simulink model "MSE452_PV_Project_Model_Student_R2018b"  (Simulink 9.2)
settings: Solver=ode45  StartTime=0.0  StopTime=0.5  MaxStep=1e-4  RelTol=1e-3
values from neighbouring files (symbols this model uses):
  Cdc = 3*Cb_solar    [MSE452_PV_Project_Model_Parameters_Student.m]    (also in MSE452_PV_Project_Model_Parameters_Studentv2.m; MSE452_PV_Project_Model_Parameters_Studentv3.m)
  Cpv = 0.05*Cb_solar    [MSE452_PV_Project_Model_Parameters_Student.m]    (also in MSE452_PV_Project_Model_Parameters_Studentv2.m; MSE452_PV_Project_Model_Parameters_Studentv3.m)
  Fb = 60    [MSE452_PV_Project_Model_Parameters_Student.m]    (also in MSE452_PV_Project_Model_Parameters_Studentv2.m; MSE452_PV_Project_Model_Parameters_Studentv3.m)
  Fs_boost = 10000    [MSE452_PV_Project_Model_Parameters_Student.m]    (also in MSE452_PV_Project_Model_Parameters_Studentv2.m; MSE452_PV_Project_Model_Parameters_Studentv3.m)
  Fsampling = 10e3    (= 10000)    [MSE452_PV_Project_Model_Parameters_Student.m]    (also in MSE452_PV_Project_Model_Parameters_Studentv2.m; MSE452_PV_Project_Model_Parameters_Studentv3.m)
  Lboost = 0.5*Lb_solar    [MSE452_PV_Project_Model_Parameters_Student.m]    (also in MSE452_PV_Project_Model_Parameters_Studentv2.m; MSE452_PV_Project_Model_Parameters_Studentv3.m)
  Lgrid = Lgrid_pu*Lb_solar    [MSE452_PV_Project_Model_Parameters_Student.m]    (also in MSE452_PV_Project_Model_Parameters_Studentv2.m; MSE452_PV_Project_Model_Parameters_Studentv3.m)
  Lgrid_pu = 0.2    [MSE452_PV_Project_Model_Parameters_Student.m]    (also in MSE452_PV_Project_Model_Parameters_Studentv2.m; MSE452_PV_Project_Model_Parameters_Studentv3.m)
  Rgrid = Rgrid_pu*Zb_solar    [MSE452_PV_Project_Model_Parameters_Student.m]    (also in MSE452_PV_Project_Model_Parameters_Studentv2.m; MSE452_PV_Project_Model_Parameters_Studentv3.m)
  Vb = 208/sqrt(3)    [MSE452_PV_Project_Model_Parameters_Student.m]    (also in MSE452_PV_Project_Model_Parameters_Studentv2.m; MSE452_PV_Project_Model_Parameters_Studentv3.m)
  Vdc_ref = sqrt(6)*(1/1)    [MSE452_PV_Project_Model_Parameters_Student.m]    (also in MSE452_PV_Project_Model_Parameters_Studentv2.m; MSE452_PV_Project_Model_Parameters_Studentv3.m = 2.44949)
undefined symbols (not defined in the file or in its folder): Rdc
undefined symbols (not defined in the file): Fs_inv, Ib_solar
libraries: powerlib x19, simulink x4, powerlib_extras x3, simulink_extras x2, re_lib x1, eePwmGenerator x1
settings Model: Creator=Student  LastModifiedBy=dw
settings SolverCC: ZeroCrossAlgorithm=Adaptive  AlgebraicLoopSolver=LineSearch
settings DataIOCC: LimitDataPoints=off  SaveFormat=Dataset  SignalLoggingSaveFormat=Dataset
settings DebuggingCC: UnderspecifiedInitializationDetection=Simplified  MergeDetectMultiDrivingBlocksExec=error  FcnCallInpInsideContextMsg=error  StateNameClashWarn=none  SFUnexpectedBacktrackingDiag=error  SFNoUnconditionalDefaultTransitionDiag=error  SFExecutionAtInitializationDiag=warning
settings HardwareCC: ProdBitPerPointer=64  ProdLargestAtomicFloat=Float  ProdIntDivRoundTo=Zero  ProdEndianess=LittleEndian  ProdHWDeviceType=Specified
settings ModelReferenceCC: PropagateSignalLabelsOutOfModel=on
settings GRTTargetCC: TargetLangStandard=C99 (ISO)  CombineOutputUpdateFcns=on  GRTInterface=off
settings ConfigComp: CovMetricSettings=dwe  CovSaveCumulativeToWorkspaceVar=off  CovSaveSingleToWorkspaceVar=off  CovExternalEMLEnable=on
settings SimscapeCC: SimscapeNormalizeSystem=off

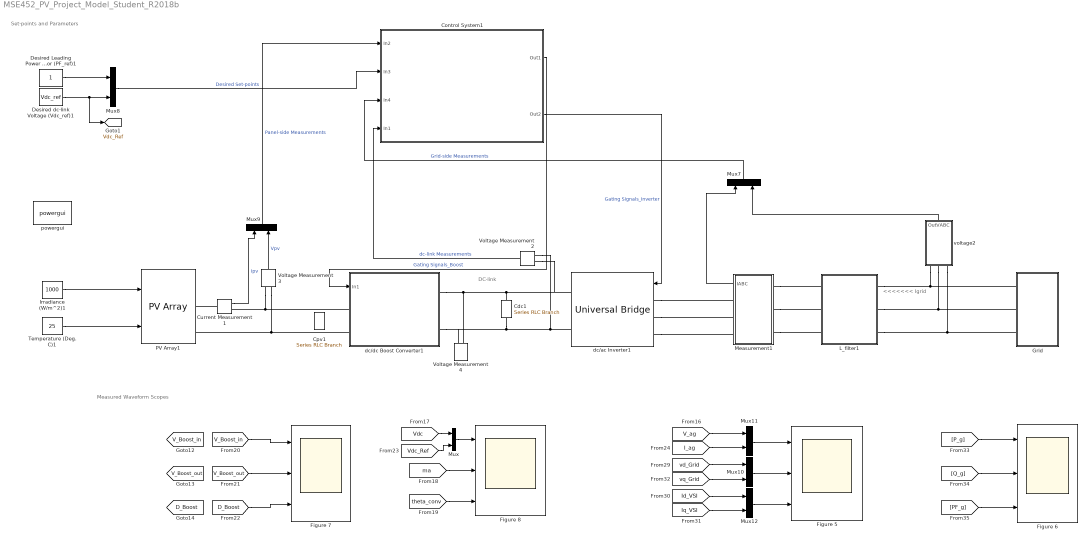
== system MSE452_PV_Project_Model_Student_R2018b ==
  note: DC-link
  note: Set-points and Parameters
  note: <<<<<<< Igrid
  note: Measured Waveform Scopes
  " voltage2" : Subsystem  mask{Base=Vb}
      mask prompts: Base "Base value"
  Cdc1 : powerlib/Elements/Series RLC Branch  LConnTagsString=__new0  RConnTagsString=__new0  BranchType=C  Resistance=Rdc  Inductance=1e-3  SetiL0=off  InitialCurrent=0  Capacitance=Cdc  Setx0=on  InitialVoltage=Vdc_capacitor_initial  Measurements=None
  Control System1 : Subsystem
  Cpv1 : powerlib/Elements/Series RLC Branch  LConnTagsString=__new0  RConnTagsString=__new0  BranchType=C  Resistance=Rdc  Inductance=1e-3  SetiL0=off  InitialCurrent=0  Capacitance=Cpv  Setx0=off  InitialVoltage=Vdc_capacitor_initial  Measurements=None
  Current Measurement1 : powerlib/Measurements/Current Measurement  PhasorSimulation=off  OutputType=Complex  PSBequivalent=0
  Desired Leading Power Factor (PF_ref)1 : Constant
  Desired dc-link Voltage (Vdc_ref)1 : Constant  Value=Vdc_ref
  Figure {5..8} (4 alike) : Scope  NumInputPorts=3
  Grid : Subsystem
  Irradiance (W/m^2)1 : Constant  Value=1000
  L_filter1 : Subsystem
  Measurement1 : Subsystem  mask{Base=Ib_solar}
      mask prompts: Base "Base value"
  Mux{,7..12} (7 alike) : Mux  Inputs=2
  PV Array1 : re_lib/Solar/PV Array  Npar=8  Nser=5  PlotType=array @ 1000 W/m2 & specified temperatures  S_vec="[ 1000 800 600 400 200  ]"  Temp_C_vec="[ 55 25  ]"  ModuleName=User-defined  PlotWhenSelected=off  Pm=229.89  Ncell=60  Voc=36.7  Isc=8.4  Vm=29.1  Im=7.9  beta_Voc_pc=-0.33899  alpha_Isc_pc=0.124  beta_Voc=-0.12441  alpha_Isc=0.010416  IL=8.4691  I0=1.485e-10  nI=0.96205  Rsh=216.9373  Rs=0.41347  RobustModel=off  RobustCellTemperature=25  BAL=off  Tc=1e-6  Tfilter=5e-5
  Temperature (Deg. C)1 : Constant  Value=25
  Voltage Measurement2 : powerlib/Measurements/Voltage Measurement  PhasorSimulation=off  OutputType=Complex  PSBequivalent=0
  Voltage Measurement3 : powerlib/Measurements/Voltage Measurement  PhasorSimulation=off  OutputType=Complex  PSBequivalent=0
  Voltage Measurement4 : powerlib/Measurements/Voltage Measurement  PhasorSimulation=off  OutputType=Complex  PSBequivalent=0
  dc/ac Inverter1 : powerlib/Power Electronics/Universal Bridge  Arms=3  SnubberResistance=1e5  SnubberCapacitance=inf  Device=IGBT / Diodes  Ron=1e-6  Lon=0  ForwardVoltages="[  0  0  ]"  ForwardVoltage=0  GTOparameters=[ 10e-6 , 20e-6 ]  IGBTparameters=[ 1e-6 , 2e-6 ]  Measurements=None  Measurements_2=None  converterType=Rectifier
  dc/dc Boost Converter1 : Subsystem
  powergui : powerlib/powergui  Priority=1  SimulationMode=Discrete  SampleTime=1e-6  frequency=60  Iterations=50  frequencyindice=0  Pbase=100e6  ErrMax=1e-4  UnitsV=kV  UnitsW=MW  buscounter=0  FunctionMessages=off  echomessages=off  EnableUseOfTLC=off  CurrentSourceSwitches=off  DisableSnubberDevices=off  DisableRonSwitches=off  DisableVfSwitches=off  DisplayEquations=off  AutomaticDiscreteSolvers=off  SolverType=Tustin  Interpol=off  ExternalGateDelay=off  methode=off  Ts=100  x0status=blocks  SPID=on  SwTol=0  HookPort=off  NonlinearTolerance=1e-4  nMaxIteration=100  ContinueOnMaxIteration=off  RestoreLinks=warning  ResistiveCurrentMeasurement=off  Frange=[0:2:500]  Ylog=off  Xlog=on  ShowGrid=off  save=off  variable=ZData  structure=0  ZoomFFT=off  StartTime=0.0  cycles=1  DisplayStyle=1  fundamental=60  FreqAxis=off  MaxFrequency=1000  frequencyindicesteady=1  RmsSteady=1  display=off
  tag scope: D_Boost=global, V_Boost_in=global, V_Boost_out=global, Vdc_Ref=global
  wires:
  [PF_g] -> Figure 6/3
  [Q_g] -> Figure 6/2
  Mux8/1 -> Control System1/2(In3)  "Desired Set-points"
  [vd_Grid] -> Mux10/1
  [V_ag] -> Mux11/1
  Control System1/1(Out1) -> dc/dc Boost Converter1/1(In1)  "Gating Signals_Boost"
  [P_g] -> Figure 6/1
  Mux/1 -> Figure 8/1
  [theta_conv] -> Figure 8/3
  Mux10/1 -> Figure 5/2
  [Id_VSI] -> Mux12/1
  Mux7/1 -> Control System1/3(In4)  "Grid-side Measurements"
  [V_Boost_out] -> Figure 7/2
  [Vdc_Ref] -> Mux/2
  Mux12/1 -> Figure 5/3
  Voltage Measurement2/1 -> Control System1/4(In1)  "dc-link Measurements"
  Desired Leading Power Factor (PF_ref)1/1 -> Mux8/1
  Irradiance (W/m^2)1/1 -> PV Array1/1
  [vq_Grid] -> Mux10/2
  [Iq_VSI] -> Mux12/2
  Mux9/1 -> Control System1/1(In2)  "Panel-side Measurements"
  Temperature (Deg. C)1/1 -> PV Array1/2
  [Vdc] -> Mux/1
  [V_Boost_in] -> Figure 7/1
  Current Measurement1/1 -> Mux9/1  "Ipv"
  [I_ag] -> Mux11/2
  [ma] -> Figure 8/2
  Mux11/1 -> Figure 5/1
  " voltage2"/1(OutVABC) -> Mux7/2
  Desired dc-link Voltage (Vdc_ref)1/1 -> [Vdc_Ref], Mux8/2
  [D_Boost] -> Figure 7/3
  Voltage Measurement3/1 -> Mux9/2  "Vpv"
  Measurement1/1(IABC) -> Mux7/1
  Control System1/2(Out2) -> dc/ac Inverter1/1  "Gating Signals_Inverter"
  connections:
  dc/dc Boost Converter1/LConn2 -- PV Array1/RConn2 -- Voltage Measurement3/LConn2
  dc/ac Inverter1/RConn2 -- Voltage Measurement2/LConn2 -- Cdc1/RConn1 -- dc/dc Boost Converter1/RConn2 -- Voltage Measurement4/LConn2
  L_filter1/LConn1 -- Grid/RConn1 -- " voltage2"/LConn1
  Voltage Measurement4/LConn1 -- dc/dc Boost Converter1/RConn1 -- Cdc1/LConn1 -- Voltage Measurement2/LConn1 -- dc/ac Inverter1/RConn1
  L_filter1/LConn3 -- Grid/RConn3 -- " voltage2"/LConn3
  L_filter1/LConn2 -- Grid/RConn2 -- " voltage2"/LConn2
  dc/dc Boost Converter1/LConn1 -- Current Measurement1/RConn1 -- Voltage Measurement3/LConn1
  Current Measurement1/LConn1 -- PV Array1/RConn1
  Measurement1/LConn3 -- L_filter1/RConn3
  Measurement1/LConn1 -- L_filter1/RConn1
  Measurement1/LConn2 -- L_filter1/RConn2
  dc/ac Inverter1/LConn1 -- Measurement1/RConn1
  dc/ac Inverter1/LConn3 -- Measurement1/RConn3
  dc/ac Inverter1/LConn2 -- Measurement1/RConn2

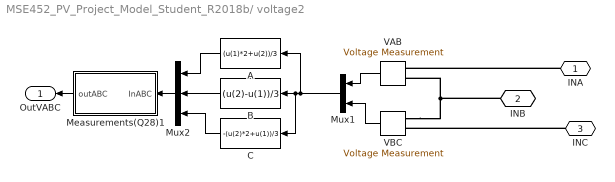
== system MSE452_PV_Project_Model_Student_R2018b/ voltage2 ==
  A : Fcn  Expr=(u(1)*2+u(2))/3
  B : Fcn  Expr=(u(2)-u(1))/3
  C : Fcn  Expr=-(u(2)*2+u(1))/3
  Measurements(Q28)1 : Subsystem  mask{Base=Base}
      mask prompts: Base "Base Value"
  Mux1 : Mux  Inputs=2
  Mux2 : Mux  Inputs=3
  VAB : powerlib/Measurements/Voltage Measurement  PhasorSimulation=off  OutputType=Complex  PSBequivalent=0
  VBC : powerlib/Measurements/Voltage Measurement  PhasorSimulation=off  OutputType=Complex  PSBequivalent=0
  INA : PMIOPort  Side=Left
  INB : PMIOPort  Port=2  Side=Left
  INC : PMIOPort  Port=3  Side=Left
  OutVABC : Outport  VectorParamsAs1DForOutWhenUnconnected=off
  wires:
  Measurements(Q28)1/1(outABC) -> OutVABC/1
  VAB/1 -> Mux1/1
  VBC/1 -> Mux1/2
  Mux1/1 -> B/1, C/1, A/1
  A/1 -> Mux2/1
  B/1 -> Mux2/2
  Mux2/1 -> Measurements(Q28)1/1(InABC)
  C/1 -> Mux2/3
  connections:
  VBC/LConn1 -- VAB/LConn2 -- INB/RConn1
  INC/RConn1 -- VBC/LConn2
  INA/RConn1 -- VAB/LConn1

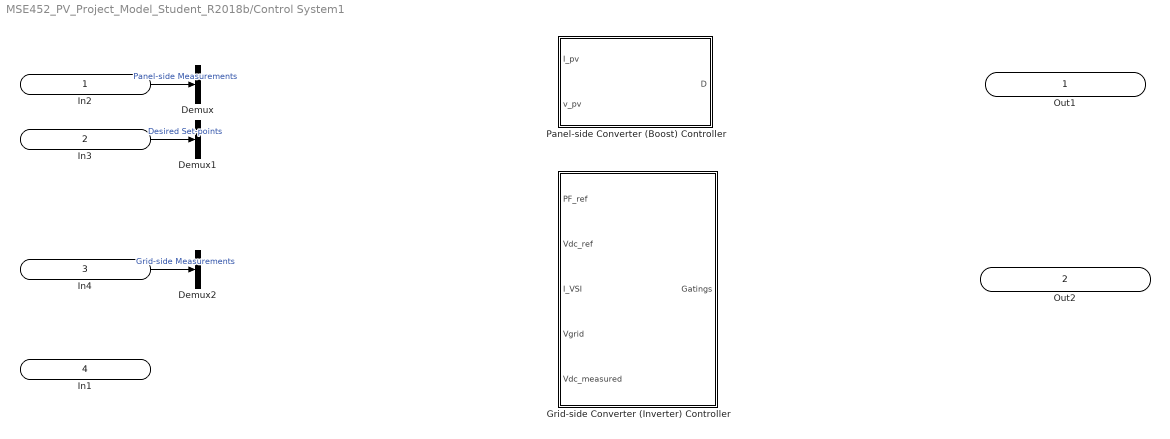
== system MSE452_PV_Project_Model_Student_R2018b/Control System1 ==
  In2 : Inport
  In3 : Inport  Port=2
  In4 : Inport  Port=3
  In1 : Inport  Port=4
  Demux : Demux  Outputs=2
  Demux1 : Demux  Outputs=2
  Demux2 : Demux  Outputs=2
  Grid-side Converter (Inverter) Controller : Subsystem
  Panel-side Converter (Boost) Controller : Subsystem
  Out1 : Outport  VectorParamsAs1DForOutWhenUnconnected=off
  Out2 : Outport  Port=2  VectorParamsAs1DForOutWhenUnconnected=off
  wires:
  In2/1 -> Demux/1  "Panel-side Measurements"
  In3/1 -> Demux1/1  "Desired Set-points"
  In4/1 -> Demux2/1  "Grid-side Measurements"

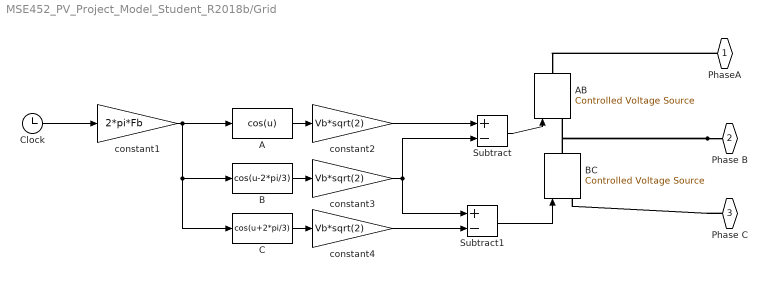
== system MSE452_PV_Project_Model_Student_R2018b/Grid ==
  A : Fcn  Expr=cos(u)
  AB : powerlib/Electrical Sources/Controlled Voltage Source  Initialize=off  Source_Type=AC  Amplitude=0  Phase=0  Frequency=0  Measurements=None
  B : Fcn  Expr=cos(u-2*pi/3)
  BC : powerlib/Electrical Sources/Controlled Voltage Source  Initialize=off  Source_Type=AC  Amplitude=0  Phase=0  Frequency=0  Measurements=None
  C : Fcn  Expr=cos(u+2*pi/3)
  Clock : Clock
  Subtract : Sum  Inputs=+-
  Subtract1 : Sum  Inputs=+-
  constant1 : Gain  Gain=2*pi*Fb
  constant2 : Gain  Gain=Vb*sqrt(2)
  constant3 : Gain  Gain=Vb*sqrt(2)
  constant4 : Gain  Gain=Vb*sqrt(2)
  PhaseA : PMIOPort  Side=Right
  Phase B : PMIOPort  Port=2  Side=Right
  Phase C : PMIOPort  Port=3  Side=Right
  wires:
  Subtract/1 -> AB/1
  Subtract1/1 -> BC/1
  A/1 -> constant2/1
  B/1 -> constant3/1
  C/1 -> constant4/1
  Clock/1 -> constant1/1
  constant1/1 -> A/1, B/1, C/1
  constant2/1 -> Subtract/1
  constant3/1 -> Subtract/2, Subtract1/1
  constant4/1 -> Subtract1/2
  connections:
  Phase B/RConn1 -- BC/RConn1 -- AB/LConn1
  PhaseA/RConn1 -- AB/RConn1
  Phase C/RConn1 -- BC/LConn1

== system MSE452_PV_Project_Model_Student_R2018b/L_filter1 ==
  Three-Phase Series RLC Branch1 : powerlib/Elements/Three-Phase Series RLC Branch  LConnTagsString=A|B|C  RConnTagsString=A|B|C  BranchType=RL  Resistance=Rgrid  Inductance=Lgrid  Capacitance=1e-6  Measurements=None
  In_A : PMIOPort  Side=Left
  out_A : PMIOPort  Port=2  Side=Right
  In_B : PMIOPort  Port=3  Side=Left
  out_B : PMIOPort  Port=4  Side=Right
  In_C : PMIOPort  Port=5  Side=Left
  out_C : PMIOPort  Port=6  Side=Right
  connections:
  In_B/RConn1 -- Three-Phase Series RLC Branch1/LConn2
  out_C/RConn1 -- Three-Phase Series RLC Branch1/RConn3
  out_B/RConn1 -- Three-Phase Series RLC Branch1/RConn2
  out_A/RConn1 -- Three-Phase Series RLC Branch1/RConn1
  Three-Phase Series RLC Branch1/LConn1 -- In_A/RConn1
  Three-Phase Series RLC Branch1/LConn3 -- In_C/RConn1

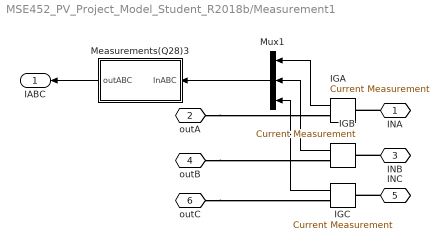
== system MSE452_PV_Project_Model_Student_R2018b/Measurement1 ==
  IGA : powerlib/Measurements/Current Measurement  PhasorSimulation=off  OutputType=Complex  PSBequivalent=0
  IGB : powerlib/Measurements/Current Measurement  PhasorSimulation=off  OutputType=Complex  PSBequivalent=0
  IGC : powerlib/Measurements/Current Measurement  PhasorSimulation=off  OutputType=Complex  PSBequivalent=0
  Measurements(Q28)3 : Subsystem  mask{Base=Base}
      mask prompts: Base "Base Value"
  Mux1 : Mux  Inputs=3
  INA : PMIOPort  Side=Left
  outA : PMIOPort  Port=2  Side=Right
  INB : PMIOPort  Port=3  Side=Left
  outB : PMIOPort  Port=4  Side=Right
  INC : PMIOPort  Port=5  Side=Left
  outC : PMIOPort  Port=6  Side=Right
  IABC : Outport  VectorParamsAs1DForOutWhenUnconnected=off
  wires:
  Measurements(Q28)3/1(outABC) -> IABC/1
  Mux1/1 -> Measurements(Q28)3/1(InABC)
  IGA/1 -> Mux1/1
  IGB/1 -> Mux1/2
  IGC/1 -> Mux1/3
  connections:
  outC/RConn1 -- IGC/RConn1
  INC/RConn1 -- IGC/LConn1
  outB/RConn1 -- IGB/RConn1
  INB/RConn1 -- IGB/LConn1
  outA/RConn1 -- IGA/RConn1
  INA/RConn1 -- IGA/LConn1

== system MSE452_PV_Project_Model_Student_R2018b/dc/dc Boost Converter1 ==
  In1 : Inport
  Diode : powerlib/Power Electronics/Diode  Ron=0.001  Lon=0  Vf=0.8  IC=0  UseSnubber=0  Rs=500  Cs=250e-9  Measurements=on
  Ideal Switch : powerlib/Power Electronics/Ideal Switch  Ron=0.001  Lon=0  IC=0  Rs=1e5  Cs=inf  Measurements=on
  L : powerlib/Elements/Series RLC Branch  LConnTagsString=__new0  RConnTagsString=__new0  BranchType=L  Resistance=Rdc  Inductance=Lboost  SetiL0=off  InitialCurrent=0  Capacitance=1e-6  Setx0=off  InitialVoltage=Vdc_capacitor_initial  Measurements=None
  PWM Generator : eePwmGenerator/PWM Generator  CarrCount=Up  Tper=1/Fs_boost  Ts=0
  In + : PMIOPort  Side=Left
  In - : PMIOPort  Port=2  Side=Left
  Out + : PMIOPort  Port=3  Side=Right
  Out - : PMIOPort  Port=4  Side=Right
  wires:
  In1/1 -> PWM Generator/1

== system MSE452_PV_Project_Model_Student_R2018b/ voltage2/Measurements(Q28)1 ==
  InABC : Inport
  Demux : Demux  Outputs=3
  Gain1 : Gain  Gain=1/Base
  Gain2 : Gain  Gain=1/Base
  Gain3 : Gain  Gain=1/Base
  Mux : Mux  Inputs=3
  outABC : Outport  VectorParamsAs1DForOutWhenUnconnected=off
  wires:
  Mux/1 -> outABC/1
  Demux/1 -> Gain2/1
  InABC/1 -> Demux/1
  Gain2/1 -> Mux/1
  Gain1/1 -> Mux/2
  Gain3/1 -> Mux/3
  Demux/2 -> Gain1/1
  Demux/3 -> Gain3/1

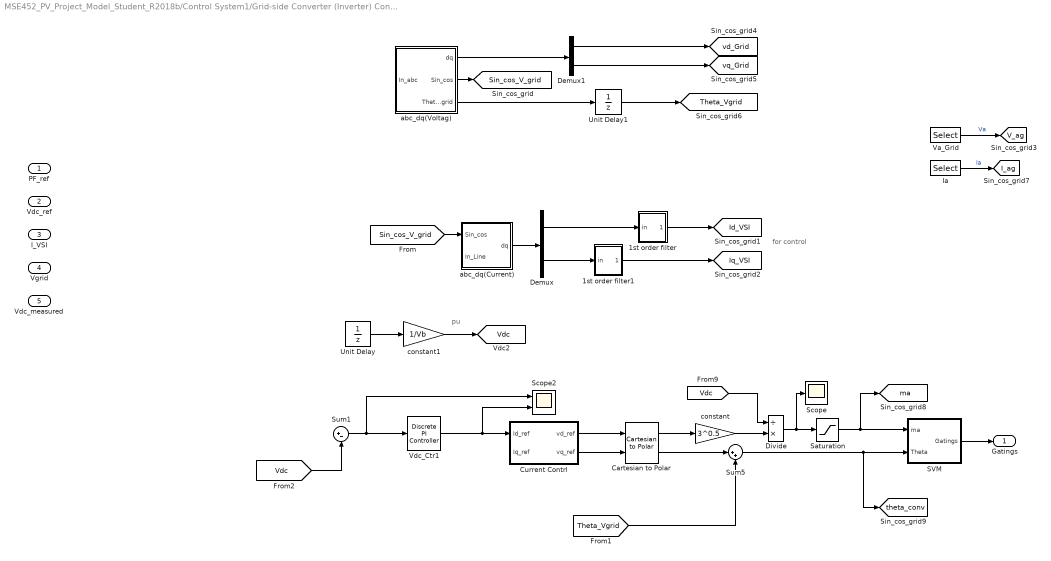
== system MSE452_PV_Project_Model_Student_R2018b/Control System1/Grid-side Converter (Inverter) Controller ==
  note: for control
  note: pu
  PF_ref : Inport
  Vdc_ref : Inport  Port=2
  I_VSI : Inport  Port=3
  Vgrid : Inport  Port=4
  Vdc_measured : Inport  Port=5
  1st order filter : Subsystem  mask{F0=500, Fs=Fsampling}
      mask prompts: F0 "Cut off Frequency"; Fs "Sampling Frequency"
  1st order filter1 : Subsystem  mask{F0=500, Fs=Fsampling}
      mask prompts: F0 "Cut off Frequency"; Fs "Sampling Frequency"
  Cartesian to Polar : simulink_extras/Transformations/Cartesian to Polar
  Current Contrl : Subsystem
  Demux : Demux  Outputs=2
  Demux1 : Demux  Outputs=2
  Divide : Product  Inputs=/*
  Ia : Selector  InputPortWidth=3  IndexOptions=Index vector (dialog)  Indices=1  OutputSizes=1
  SVM : Subsystem  mask{Fs=Fs_inv}
      mask prompts: Fs "Switching frequency"
  Saturation : Saturate  UpperLimit=1  LowerLimit=0  SampleTime=1/Fsampling
  Scope : Scope
  Scope2 : Scope  NumInputPorts=2
  Sum1 : Sum  Inputs=|+-
  Sum5 : Sum  Inputs=|++
  Unit Delay : UnitDelay  InitialCondition=Vb*3^0.5  SampleTime=1/Fsampling  HasFrameUpgradeWarning=on
  Unit Delay1 : UnitDelay  InitialCondition=Vb*3^0.5  SampleTime=1/Fsampling  HasFrameUpgradeWarning=on
  Va_Grid : Selector  InputPortWidth=3  IndexOptions=Index vector (dialog)  Indices=1  OutputSizes=1
  Vdc_Ctr1 : powerlib_extras/Discrete  Control Blocks/Discrete PI Controller  Kp=1  Ki=200  Par_Limits=[1.5 -1.5]  Init=0  Ts=1/Fsampling
  abc_dq(Current) : Subsystem
  abc_dq(Voltag) : Subsystem
  constant : Gain  Gain=3^0.5
  constant1 : Gain  Gain=1/Vb
  Gatings : Outport  VectorParamsAs1DForOutWhenUnconnected=off
  tag scope: I_ag=global, Id_VSI=global, Iq_VSI=global, Sin_cos_V_grid=global, Theta_Vgrid=global, V_ag=global, Vdc=global, ma=global, theta_conv=global, vd_Grid=global, vq_Grid=global
  wires:
  Demux/1 -> 1st order filter/1(in)
  Current Contrl/1(vd_ref) -> Cartesian to Polar/1
  1st order filter1/1(Out) -> [Iq_VSI]
  [Theta_Vgrid] -> Sum5/2
  Saturation/1 -> [ma], SVM/1(ma)
  abc_dq(Voltag)/2(Sin_cos) -> [Sin_cos_V_grid]
  Unit Delay/1 -> constant1/1
  Divide/1 -> Scope/1, Saturation/1
  Ia/1 -> [I_ag]  "Ia"
  Cartesian to Polar/1 -> constant/1
  constant/1 -> Divide/2
  [Vdc] -> Divide/1
  Demux1/2 -> [vq_Grid]
  abc_dq(Current)/1(dq) -> Demux/1
  constant1/1 -> [Vdc]
  Demux/2 -> 1st order filter1/1(in)
  SVM/1(Gatings) -> Gatings/1
  Va_Grid/1 -> [V_ag]  "Va"
  abc_dq(Voltag)/1(dq) -> Demux1/1
  Current Contrl/2(vq_ref) -> Cartesian to Polar/2
  1st order filter/1(Out) -> [Id_VSI]
  Cartesian to Polar/2 -> Sum5/1
  Sum5/1 -> [theta_conv], SVM/2(Theta)
  abc_dq(Voltag)/3(Theta_Vgrid) -> Unit Delay1/1
  [Sin_cos_V_grid] -> abc_dq(Current)/1(Sin_cos)
  Demux1/1 -> [vd_Grid]
  Unit Delay1/1 -> [Theta_Vgrid]
  [Vdc] -> Sum1/2
  Sum1/1 -> Scope2/1, Vdc_Ctr1/1
  Vdc_Ctr1/1 -> Scope2/2, Current Contrl/1(Id_ref)

== system MSE452_PV_Project_Model_Student_R2018b/Control System1/Panel-side Converter (Boost) Controller ==
  I_pv : Inport
  v_pv : Inport  Port=2
  P & O : Subsystem
  PID Controller : simulink/Continuous/PID Controller  Controller=PI  Form=Parallel  TimeDomain=Continuous-time  SampleTime=-1  IntegratorMethod=Forward Euler  FilterMethod=Forward Euler  ControllerParametersSource=internal  P=-0.01  I=-0.03  D=0  UseFilter=on  N=100  TunerSelectOption=Transfer Function Based (PID Tuner App)  InitialConditionSource=internal  InitialConditionForIntegrator=0  InitialConditionForFilter=0  DifferentiatorICPrevScaledInput=0  ExternalReset=none  TrackingMode=off  Kt=1  LimitOutput=off  UpperSaturationLimit=inf  LowerSaturationLimit=-inf  LinearizeAsGain=on  AntiWindupMode=none  Kb=1  POutMin=[]  POutMax=[]  IOutMin=[]  IOutMax=[]  DOutMin=[]  DOutMax=[]  NOutMin=[]  NOutMax=[]  SumOutMin=[]  SumOutMax=[]  SaturationOutMin=[]  SaturationOutMax=[]  PParamMin=[]  PParamMax=[]  IParamMin=[]  IParamMax=[]  DParamMin=[]  DParamMax=[]  NParamMin=[]  NParamMax=[]  KbParamMin=[]  KbParamMax=[]  KtParamMin=[]  KtParamMax=[]  KbOutMin=[]  KbOutMax=[]  KtOutMin=[]  KtOutMax=[]  IntegratorOutMin=[]  IntegratorOutMax=[]  FilterOutMin=[]  FilterOutMax=[]  SumI1OutMin=[]  SumI1OutMax=[]  SumI2OutMin=[]  SumI2OutMax=[]  SumI3OutMin=[]  SumI3OutMax=[]  SumI4OutMin=[]  SumI4OutMax=[]  SumDOutMin=[]  SumDOutMax=[]  DifferentiatorOutMin=[]  DifferentiatorOutMax=[]  FilterDiffOutCoefMin=[]  FilterDiffOutCoefMax=[]  ReciprocalOutMin=[]  ReciprocalOutMax=[]  SumDenOutMin=[]  SumDenOutMax=[]  SumNumOutMin=[]  SumNumOutMax=[]  DivideOutMin=[]  DivideOutMax=[]  IntegratorContinuousStateAttributes=''  IntegratorStateMustResolveToSignalObject=off  IntegratorRTWStateStorageClass=Auto  FilterContinuousStateAttributes=''  FilterStateMustResolveToSignalObject=off  FilterRTWStateStorageClass=Auto  ParallelPVariant=InternalParameters  IdealPVariant=Disabled  IVariant=InternalParameters  DVariant=Disabled  IntegratorVariant=Continuous  SatVariant=Disabled  AWVariant=Passthrough  PCopyVariant=Disabled  TRVariant=Disabled  FdbkBlocksVariant=Forward  IdealPFdbkVariant=Disabled  SatFdbkVariant=Disabled  DerivativeFilterVariant=Disabled  NVariant=Disabled  NCopyVariant=Disabled_SignalSpec  FilterICVariant=Disabled  IntegratorICVariant=InternalICs  ExternalResetVariant=Disabled  TRSumVariant=Passthrough  SumFdbkVariant=Disabled  SumVariant=Sum_PI
  Saturation : Saturate  UpperLimit=1  LowerLimit=0
  Sum1 : Sum  Inputs=|+-
  D : Outport  VectorParamsAs1DForOutWhenUnconnected=off
  wires:
  Sum1/1 -> PID Controller/1
  v_pv/1 -> Sum1/2  "Vpv"
  P & O/1(Vmpp) -> Sum1/1
  PID Controller/1 -> Saturation/1
  Saturation/1 -> D/1

== system MSE452_PV_Project_Model_Student_R2018b/Measurement1/Measurements(Q28)3 ==
  InABC : Inport
  Demux : Demux  Outputs=3
  Gain1 : Gain  Gain=1/Base
  Gain2 : Gain  Gain=1/Base
  Gain3 : Gain  Gain=1/Base
  Mux : Mux  Inputs=3
  outABC : Outport  VectorParamsAs1DForOutWhenUnconnected=off
  wires:
  Mux/1 -> outABC/1
  Demux/1 -> Gain2/1
  InABC/1 -> Demux/1
  Gain2/1 -> Mux/1
  Gain1/1 -> Mux/2
  Gain3/1 -> Mux/3
  Demux/2 -> Gain1/1
  Demux/3 -> Gain3/1

== system MSE452_PV_Project_Model_Student_R2018b/Control System1/Grid-side Converter (Inverter) Controller/1st order filter ==
  in : Inport
  Discrete Transfer 1Hz3 : DiscreteTransferFcn  Numerator=[1/Fs*(2*pi*F0) 1/Fs*(2*pi*F0) ]  Denominator="[((2*pi*F0)/Fs+2)  ((2*pi*F0)/Fs-2)]"  SampleTime=1/Fs
  Out : Outport  VectorParamsAs1DForOutWhenUnconnected=off
  wires:
  Discrete Transfer 1Hz3/1 -> Out/1
  in/1 -> Discrete Transfer 1Hz3/1

== system MSE452_PV_Project_Model_Student_R2018b/Control System1/Grid-side Converter (Inverter) Controller/1st order filter1 ==
  in : Inport
  Discrete Transfer 1Hz3 : DiscreteTransferFcn  Numerator=[1/Fs*(2*pi*F0) 1/Fs*(2*pi*F0) ]  Denominator="[((2*pi*F0)/Fs+2)  ((2*pi*F0)/Fs-2)]"  SampleTime=1/Fs
  Out : Outport  VectorParamsAs1DForOutWhenUnconnected=off
  wires:
  in/1 -> Discrete Transfer 1Hz3/1
  Discrete Transfer 1Hz3/1 -> Out/1

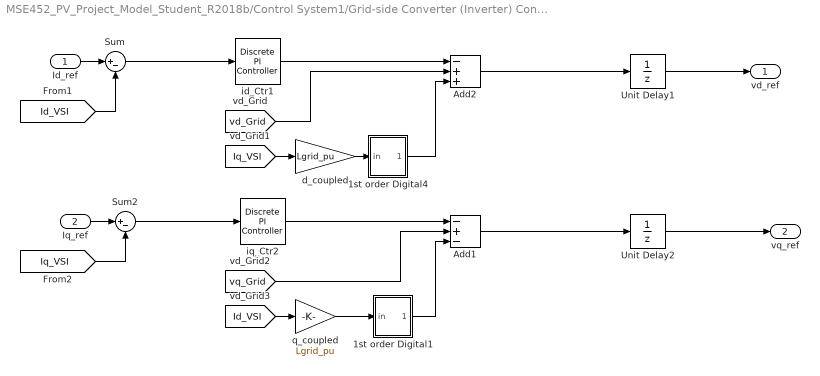
== system MSE452_PV_Project_Model_Student_R2018b/Control System1/Grid-side Converter (Inverter) Controller/Current Contrl ==
  Id_ref : Inport
  Iq_ref : Inport  Port=2
  1st order Digital1 : Subsystem  mask{F0=10, Fs=Fsampling}
      mask prompts: F0 "Cut off Frequency"; Fs "Sampling Frequency"
  1st order Digital4 : Subsystem  mask{F0=10, Fs=Fsampling}
      mask prompts: F0 "Cut off Frequency"; Fs "Sampling Frequency"
  Add1 : Sum  Inputs=-+-
  Add2 : Sum  Inputs=-++
  Sum : Sum  Inputs=|+-
  Sum2 : Sum  Inputs=|+-
  Unit Delay1 : UnitDelay  SampleTime=1/Fsampling  HasFrameUpgradeWarning=on
  Unit Delay2 : UnitDelay  SampleTime=1/Fsampling  HasFrameUpgradeWarning=on
  d_coupled : Gain  Gain=Lgrid_pu
  id_Ctr1 : powerlib_extras/Discrete  Control Blocks/Discrete PI Controller  Kp=0.3  Ki=200  Par_Limits=[1 -1]  Init=0  Ts=1/Fsampling
  iq_Ctr2 : powerlib_extras/Discrete  Control Blocks/Discrete PI Controller  Kp=0.3  Ki=200  Par_Limits=[1 -1]  Init=0  Ts=1/Fsampling
  q_coupled : Gain  Gain=Lgrid_pu
  vd_ref : Outport  VectorParamsAs1DForOutWhenUnconnected=off
  vq_ref : Outport  Port=2  VectorParamsAs1DForOutWhenUnconnected=off
  wires:
  id_Ctr1/1 -> Add2/1
  [vd_Grid] -> Add2/2
  [Iq_VSI] -> d_coupled/1
  Sum/1 -> id_Ctr1/1
  iq_Ctr2/1 -> Add1/1
  [vq_Grid] -> Add1/2
  [Id_VSI] -> q_coupled/1
  Sum2/1 -> iq_Ctr2/1
  [Id_VSI] -> Sum/2
  [Iq_VSI] -> Sum2/2
  Id_ref/1 -> Sum/1
  Add2/1 -> Unit Delay1/1
  Iq_ref/1 -> Sum2/1
  Add1/1 -> Unit Delay2/1
  d_coupled/1 -> 1st order Digital4/1(in)
  q_coupled/1 -> 1st order Digital1/1(in)
  1st order Digital4/1(Out) -> Add2/3
  1st order Digital1/1(Out) -> Add1/3
  Unit Delay2/1 -> vq_ref/1
  Unit Delay1/1 -> vd_ref/1

== system MSE452_PV_Project_Model_Student_R2018b/Control System1/Grid-side Converter (Inverter) Controller/SVM ==
  ma : Inport
  Theta : Inport  Port=2
  Pulses : Subsystem
  Sector judge : Subsystem
  Ta Tb T0 Calculation : Subsystem
  Ts : Constant  Value=1/Fs
  Zero-Order Hold : ZeroOrderHold  SampleTime=1/(2*Fs)
  Zero-Order Hold1 : ZeroOrderHold  SampleTime=1/(2*Fs)
  Gatings : Outport  VectorParamsAs1DForOutWhenUnconnected=off
  wires:
  Ta Tb T0 Calculation/3(T0) -> Pulses/4(T0)
  Ts/1 -> Ta Tb T0 Calculation/3(Ts)
  Ta Tb T0 Calculation/1(Ta1) -> Pulses/2(Ta1)
  Ta Tb T0 Calculation/2(Tb1) -> Pulses/3(Tb1)
  Sector judge/1(Sector) -> Pulses/1(Sector)
  Sector judge/2(Cal_theta) -> Ta Tb T0 Calculation/1(Cal_theta)
  Theta/1 -> Zero-Order Hold1/1
  Pulses/1(Gating) -> Gatings/1
  ma/1 -> Zero-Order Hold/1
  Zero-Order Hold/1 -> Ta Tb T0 Calculation/2(ma)
  Zero-Order Hold1/1 -> Sector judge/1(theta)

== system MSE452_PV_Project_Model_Student_R2018b/Control System1/Grid-side Converter (Inverter) Controller/abc_dq(Current) ==
  Sin_cos : Inport
  In_Line : Inport  Port=2
  Beta : Fcn  Expr=(2/3)*(u(1)*0+u(2)*(3^0.5/2)+u(3)*(-3^0.5/2))
  Mux1 : Mux  Inputs=2
  Mux4 : Mux  Inputs=2
  Mux6 : Mux  Inputs=2
  alpha : Fcn  Expr=(2/3)*(u(1)*1+u(2)*(-1/2)+u(3)*(-1/2))
  d1 : Fcn  Expr=u(2)*u(4)+u(1)*u(3)
  q1 : Fcn  Expr=-u(2)*u(3)+u(1)*u(4)
  dq : Outport  VectorParamsAs1DForOutWhenUnconnected=off
  wires:
  Sin_cos/1 -> Mux4/2
  Beta/1 -> Mux1/1
  alpha/1 -> Mux1/2
  Mux1/1 -> Mux4/1
  In_Line/1 -> Beta/1, alpha/1
  Mux4/1 -> q1/1, d1/1
  d1/1 -> Mux6/1
  q1/1 -> Mux6/2
  Mux6/1 -> dq/1

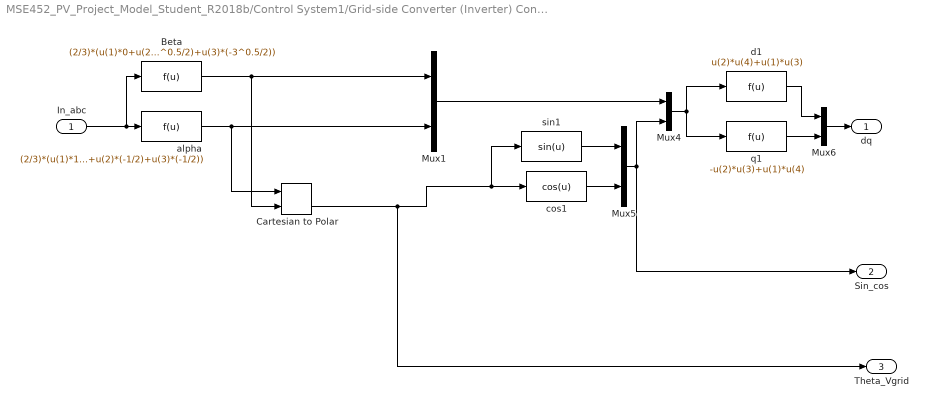
== system MSE452_PV_Project_Model_Student_R2018b/Control System1/Grid-side Converter (Inverter) Controller/abc_dq(Voltag) ==
  In_abc : Inport
  Beta : Fcn  Expr=(2/3)*(u(1)*0+u(2)*(3^0.5/2)+u(3)*(-3^0.5/2))
  Cartesian to Polar : simulink_extras/Transformations/Cartesian to Polar
  Mux{1,4..6} (4 alike) : Mux  Inputs=2
  alpha : Fcn  Expr=(2/3)*(u(1)*1+u(2)*(-1/2)+u(3)*(-1/2))
  cos1 : Fcn  Expr=cos(u)
  d1 : Fcn  Expr=u(2)*u(4)+u(1)*u(3)
  q1 : Fcn  Expr=-u(2)*u(3)+u(1)*u(4)
  sin1 : Fcn  Expr=sin(u)
  dq : Outport  VectorParamsAs1DForOutWhenUnconnected=off
  Sin_cos : Outport  Port=2  VectorParamsAs1DForOutWhenUnconnected=off
  Theta_Vgrid : Outport  Port=3  VectorParamsAs1DForOutWhenUnconnected=off
  wires:
  Mux6/1 -> dq/1
  q1/1 -> Mux6/2
  d1/1 -> Mux6/1
  cos1/1 -> Mux5/2
  sin1/1 -> Mux5/1
  Mux4/1 -> d1/1, q1/1
  In_abc/1 -> alpha/1, Beta/1
  Mux1/1 -> Mux4/1
  alpha/1 -> Cartesian to Polar/1, Mux1/2
  Beta/1 -> Cartesian to Polar/2, Mux1/1
  Mux5/1 -> Mux4/2, Sin_cos/1
  Cartesian to Polar/2 -> Theta_Vgrid/1, cos1/1, sin1/1

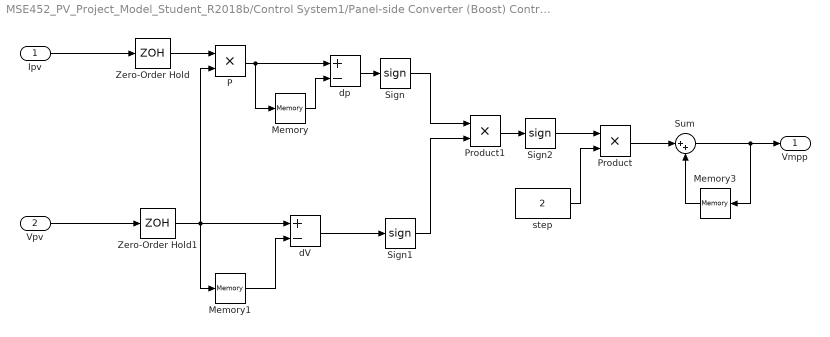
== system MSE452_PV_Project_Model_Student_R2018b/Control System1/Panel-side Converter (Boost) Controller/P & O ==
  Ipv : Inport
  Vpv : Inport  Port=2
  Memory : Memory  InheritSampleTime=on
  Memory1 : Memory  InheritSampleTime=on
  Memory3 : Memory  InheritSampleTime=on
  P : Product  RndMeth=Zero
  Product : Product  RndMeth=Zero
  Product1 : Product  RndMeth=Zero
  Sign : Signum
  Sign1 : Signum
  Sign2 : Signum
  Sum : Sum  Inputs=|++
  Zero-Order Hold : ZeroOrderHold  SampleTime=0.002
  Zero-Order Hold1 : ZeroOrderHold  SampleTime=0.002
  dV : Sum  Inputs=+-
  dp : Sum  Inputs=+-
  step : Constant  Value=2
  Vmpp : Outport  VectorParamsAs1DForOutWhenUnconnected=off
  wires:
  Memory1/1 -> dV/2
  Memory/1 -> dp/2
  Vpv/1 -> Zero-Order Hold1/1
  dV/1 -> Sign1/1
  step/1 -> Product/2
  Product/1 -> Sum/1
  Sign/1 -> Product1/1
  Sign1/1 -> Product1/2
  Product1/1 -> Sign2/1
  Ipv/1 -> Zero-Order Hold/1
  Zero-Order Hold1/1 -> dV/1, Memory1/1, P/2
  Zero-Order Hold/1 -> P/1
  P/1 -> Memory/1, dp/1
  dp/1 -> Sign/1
  Sign2/1 -> Product/1
  Sum/1 -> Memory3/1, Vmpp/1
  Memory3/1 -> Sum/2

== system MSE452_PV_Project_Model_Student_R2018b/Control System1/Grid-side Converter (Inverter) Controller/Current Contrl/1st order Digital1 ==
  in : Inport
  Discrete Transfer 1Hz3 : DiscreteTransferFcn  Numerator=[1/Fs*(2*pi*F0) 1/Fs*(2*pi*F0) ]  Denominator="[((2*pi*F0)/Fs+2)  ((2*pi*F0)/Fs-2)]"  SampleTime=1/Fs
  Out : Outport  VectorParamsAs1DForOutWhenUnconnected=off
  wires:
  in/1 -> Discrete Transfer 1Hz3/1
  Discrete Transfer 1Hz3/1 -> Out/1

== system MSE452_PV_Project_Model_Student_R2018b/Control System1/Grid-side Converter (Inverter) Controller/Current Contrl/1st order Digital4 ==
  in : Inport
  Discrete Transfer 1Hz3 : DiscreteTransferFcn  Numerator=[1/Fs*(2*pi*F0) 1/Fs*(2*pi*F0) ]  Denominator="[((2*pi*F0)/Fs+2)  ((2*pi*F0)/Fs-2)]"  SampleTime=1/Fs
  Out : Outport  VectorParamsAs1DForOutWhenUnconnected=off
  wires:
  Discrete Transfer 1Hz3/1 -> Out/1
  in/1 -> Discrete Transfer 1Hz3/1

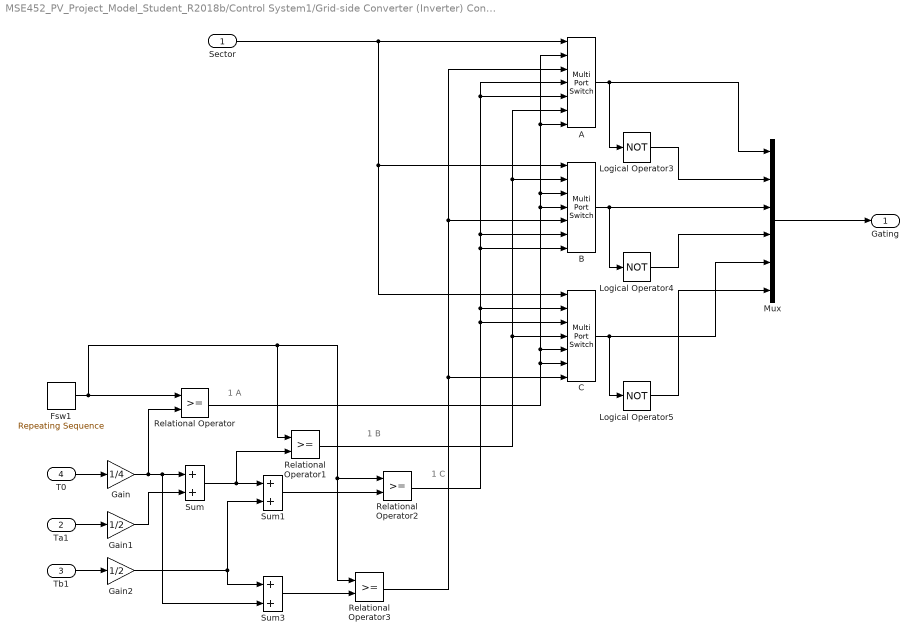
== system MSE452_PV_Project_Model_Student_R2018b/Control System1/Grid-side Converter (Inverter) Controller/SVM/Pulses ==
  note: 1 A
  note: 1 B
  note: 1 C
  Sector : Inport
  Ta1 : Inport  Port=2
  Tb1 : Inport  Port=3
  T0 : Inport  Port=4
  A : MultiPortSwitch  Inputs=6
  B : MultiPortSwitch  Inputs=6
  C : MultiPortSwitch  Inputs=6
  Fsw1 : simulink/Sources/Repeating Sequence  rep_seq_t=[0 1/Fs/2 1/Fs]  rep_seq_y=[0 1/Fs/2 0]
  Gain : Gain  Gain=1/4
  Gain1 : Gain  Gain=1/2
  Gain2 : Gain  Gain=1/2
  Logical Operator3 : Logic  Operator=NOT  AllPortsSameDT=off
  Logical Operator4 : Logic  Operator=NOT  AllPortsSameDT=off
  Logical Operator5 : Logic  Operator=NOT  AllPortsSameDT=off
  Mux : Mux  Inputs=6
  Relational Operator{,1..3} (4 alike) : RelationalOperator  OutDataTypeStr=boolean  RndMeth=Nearest
  Sum : Sum
  Sum1 : Sum
  Sum3 : Sum
  Gating : Outport  VectorParamsAs1DForOutWhenUnconnected=off
  wires:
  T0/1 -> Gain/1
  Ta1/1 -> Gain1/1
  Tb1/1 -> Gain2/1
  Gain/1 -> Relational Operator/2, Sum/1, Sum3/2
  Gain1/1 -> Sum/2
  Gain2/1 -> Sum1/2, Sum3/1
  Sum/1 -> Sum1/1, Relational Operator1/2
  Fsw1/1 -> Relational Operator/1, Relational Operator1/1, Relational Operator2/1, Relational Operator3/1
  Sum1/1 -> Relational Operator2/2
  Sector/1 -> A/1, C/1, B/1
  A/1 -> Logical Operator3/1, Mux/1
  B/1 -> Logical Operator4/1, Mux/3
  C/1 -> Logical Operator5/1, Mux/5
  Relational Operator/1 -> A/2, A/7, B/3, B/4, C/5, C/6
  Relational Operator1/1 -> C/4, B/2, A/6
  Relational Operator2/1 -> B/7, A/4, A/5, B/6, C/2, C/3
  Mux/1 -> Gating/1
  Logical Operator3/1 -> Mux/2
  Logical Operator4/1 -> Mux/4
  Logical Operator5/1 -> Mux/6
  Sum3/1 -> Relational Operator3/2
  Relational Operator3/1 -> A/3, B/5, C/7

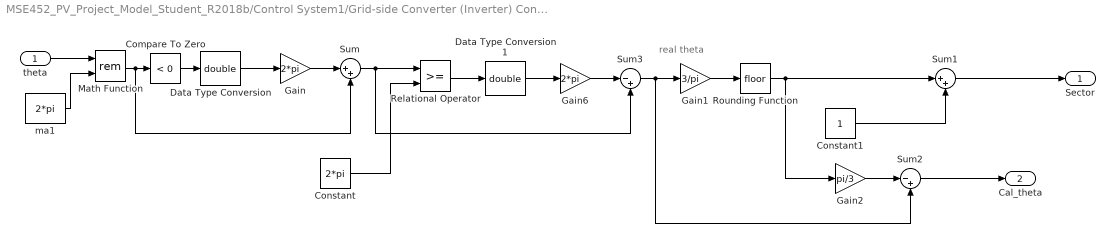
== system MSE452_PV_Project_Model_Student_R2018b/Control System1/Grid-side Converter (Inverter) Controller/SVM/Sector judge ==
  note: real theta
  theta : Inport
  Compare To Zero : simulink/Logic and Bit Operations/Compare To Zero  relop=<  OutDataTypeStr=uint8  ZeroCross=off
  Constant : Constant  Value=2*pi
  Constant1 : Constant  OutDataTypeStr=boolean
  Data Type Conversion : DataTypeConversion  OutDataTypeStr=double
  Data Type Conversion1 : DataTypeConversion  OutDataTypeStr=double
  Gain : Gain  Gain=2*pi
  Gain1 : Gain  Gain=3/pi
  Gain2 : Gain  Gain=pi/3
  Gain6 : Gain  Gain=2*pi
  Math Function : Math  Operator=rem  SaturateOnIntegerOverflow=on
  Relational Operator : RelationalOperator  OutDataTypeStr=boolean  RndMeth=Nearest
  Rounding Function : Rounding
  Sum : Sum  Inputs=|++
  Sum1 : Sum  Inputs=|++  SaturateOnIntegerOverflow=on
  Sum2 : Sum  Inputs=|-+
  Sum3 : Sum  Inputs=|-+
  ma1 : Constant  Value=2*pi
  Sector : Outport  VectorParamsAs1DForOutWhenUnconnected=off
  Cal_theta : Outport  Port=2  VectorParamsAs1DForOutWhenUnconnected=off
  wires:
  Math Function/1 -> Compare To Zero/1, Sum/2
  Compare To Zero/1 -> Data Type Conversion/1
  Data Type Conversion/1 -> Gain/1
  Gain/1 -> Sum/1
  Gain1/1 -> Rounding Function/1
  Rounding Function/1 -> Sum1/1, Gain2/1
  Sum1/1 -> Sector/1
  Constant1/1 -> Sum1/2
  Gain2/1 -> Sum2/1
  Sum2/1 -> Cal_theta/1
  Sum/1 -> Relational Operator/1, Sum3/2
  Constant/1 -> Relational Operator/2
  Relational Operator/1 -> Data Type Conversion1/1
  Data Type Conversion1/1 -> Gain6/1
  Gain6/1 -> Sum3/1
  Sum3/1 -> Gain1/1, Sum2/2
  ma1/1 -> Math Function/2
  theta/1 -> Math Function/1

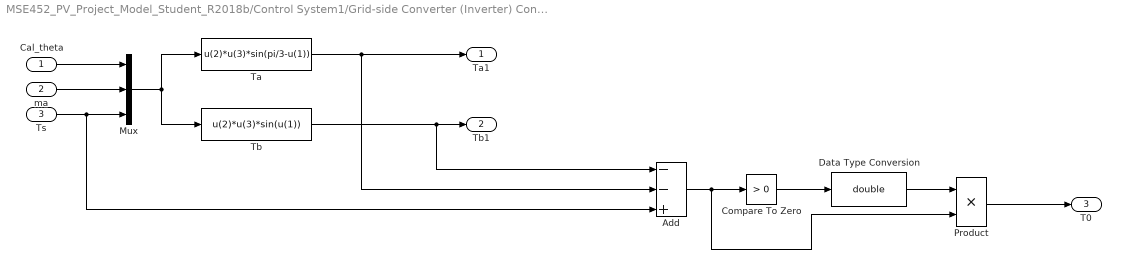
== system MSE452_PV_Project_Model_Student_R2018b/Control System1/Grid-side Converter (Inverter) Controller/SVM/Ta Tb T0 Calculation ==
  Cal_theta : Inport
  ma : Inport  Port=2
  Ts : Inport  Port=3
  Add : Sum  Inputs=--+
  Compare To Zero : simulink/Logic and Bit Operations/Compare To Zero  relop=>  OutDataTypeStr=boolean
  Data Type Conversion : DataTypeConversion  OutDataTypeStr=double
  Mux : Mux  Inputs=3
  Product : Product  RndMeth=Zero
  Ta : Fcn  Expr=u(2)*u(3)*sin(pi/3-u(1))
  Tb : Fcn  Expr=u(2)*u(3)*sin(u(1))
  Ta1 : Outport  VectorParamsAs1DForOutWhenUnconnected=off
  Tb1 : Outport  Port=2  VectorParamsAs1DForOutWhenUnconnected=off
  T0 : Outport  Port=3  VectorParamsAs1DForOutWhenUnconnected=off
  wires:
  Ts/1 -> Mux/3, Add/3
  ma/1 -> Mux/2
  Cal_theta/1 -> Mux/1
  Mux/1 -> Ta/1, Tb/1
  Ta/1 -> Add/2, Ta1/1
  Product/1 -> T0/1
  Tb/1 -> Tb1/1, Add/1
  Add/1 -> Compare To Zero/1, Product/2
  Compare To Zero/1 -> Data Type Conversion/1
  Data Type Conversion/1 -> Product/1
